simulink model "GSM_TX"  (R2022b)
settings: Solver=ode45  StartTime=0.0  StopTime=inf  RelTol=1e-3  EnableMultiTasking=on
libraries: dsparch4 x2, commanapbnd3 x2
settings Model: Creator=Kyrillos  LastModifiedBy=anand
settings SolverCC: AlgebraicLoopSolver=TrustRegion
settings DataIOCC: LimitDataPoints=on  SaveFormat=Array  InspectSignalLogs=on  ReturnWorkspaceOutputs=off
settings OptimizationCC: LifeSpan=inf
settings DebuggingCC: SolverPrmCheckMsg=warning  UnconnectedInputMsg=warning  UnconnectedOutputMsg=warning  UnconnectedLineMsg=warning  SFUnexpectedBacktrackingDiag=warning  SFNoUnconditionalDefaultTransitionDiag=warning  SFExecutionAtInitializationDiag=none  SFMachineParentedDataDiag=warning  ArithmeticOperatorsInVariantConditions=warning
settings HardwareCC: ProdBitPerPointer=32  ProdBitPerSizeT=32  ProdBitPerPtrDiffT=32  ProdLargestAtomicFloat=None  ProdIntDivRoundTo=Undefined  ProdEndianess=Unspecified  ProdWordSize=32  ProdHWDeviceType=32-bit Generic
settings ModelReferenceCC: PropagateSignalLabelsOutOfModel=off
settings SFSimCC: SimUseLocalCustomCode=off  CustomCodeUndefinedFunction=UseInterfaceOnly
settings RTWCC: RTWUseLocalCustomCode=off
settings CodeAppCC: StateflowObjectComments=on
settings GRTTargetCC: TargetLangStandard=C89/C90 (ANSI)
settings ConfigComp: CovMetricSettings=dw  CovSaveCumulativeToWorkspaceVar=on  CovSaveSingleToWorkspaceVar=on  CovExternalEMLEnable=off  CovSFcnEnable=off
settings ConfigurationSet: Description=SimMechanics 2G

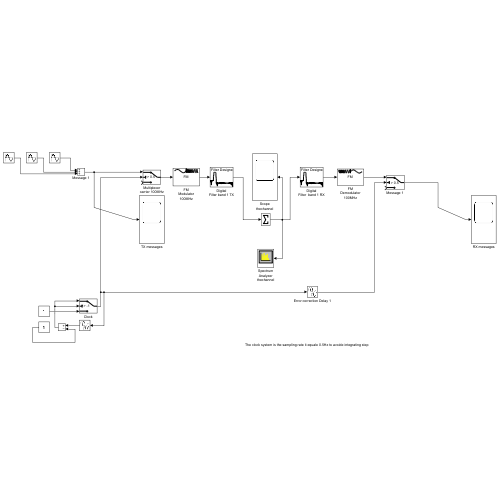
[thumbnail: Simulink's stored preview of the top-level diagram]
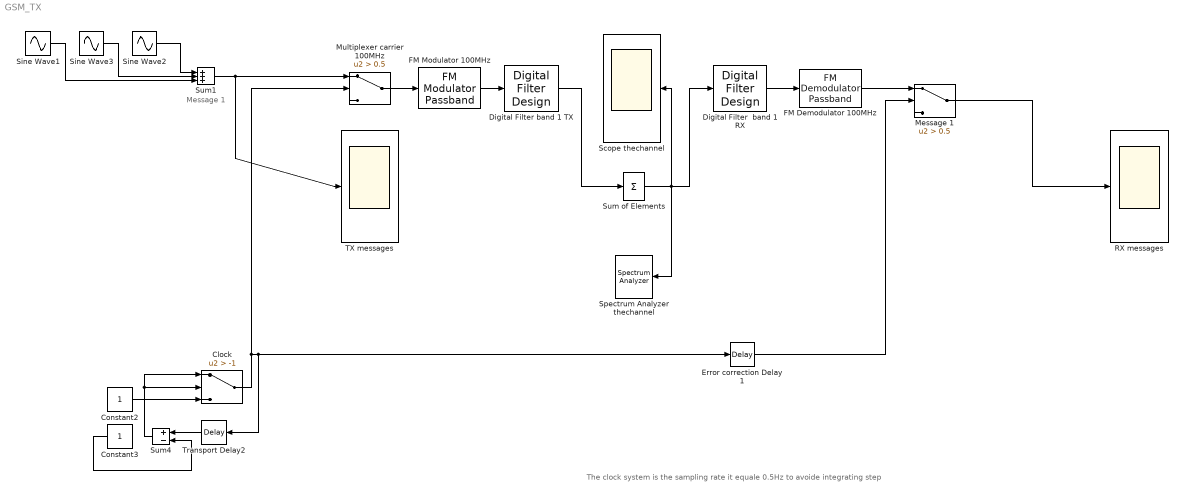
== system GSM_TX ==
  note: The clock system is the sampling rate it equale 0.5Hz to avoide integrating step
  note: Message 1
  Clock : Switch  Criteria=u2 > Threshold  Threshold=-1  SampleTime=0.001  SaturateOnIntegerOverflow=off  InputSameDT=off
  Constant2 : Constant
  Constant3 : Constant
  Digital Filter  band 1 RX : dsparch4/Digital Filter Design  mwdsp_browser_bugfix_var=off
  Digital Filter band 1 TX : dsparch4/Digital Filter Design  mwdsp_browser_bugfix_var=off
  Error correction Delay 1 : TransportDelay  DelayTime=0.3
  FM Demodulator 100MHz : commanapbnd3/FM Demodulator Passband  Fc=100  Ph=0  Kc=0.2  Ho=100
  FM Modulator 100MHz : commanapbnd3/FM Modulator Passband  Fc=100  Ph=0  Kc=0.2
  "Message 1 " : Switch  Criteria=u2 > Threshold  Threshold=0.5  SampleTime=0.001  SaturateOnIntegerOverflow=off  InputSameDT=off
  Multiplexer carrier 100MHz : Switch  Criteria=u2 > Threshold  Threshold=0.5  SampleTime=0.001  SaturateOnIntegerOverflow=off  InputSameDT=off
  RX messages : Scope
      settings: Priority=3
  Scope thechannel : Scope
      settings: Priority=3
  Sine Wave1 : Sin  Amplitude=10/5  Frequency=10*pi  SampleTime=0.001
  Sine Wave2 : Sin  Amplitude=10  Frequency=2*pi  SampleTime=0.001
  Sine Wave3 : Sin  Amplitude=10/3  Frequency=6*pi  SampleTime=0.001
  Spectrum Analyzer thechannel : SpectrumAnalyzer
  Sum of Elements : Sum  Inputs=+  SampleTime=0.001
  Sum1 : Sum  Inputs=+++
  Sum4 : Sum  Inputs=+-
  TX messages : Scope
      settings: Priority=3
  Transport Delay2 : TransportDelay
  wires:
  Sum1/1 -> Multiplexer carrier 100MHz/1, TX messages/1
  Multiplexer carrier 100MHz/1 -> FM Modulator 100MHz/1
  Digital Filter  band 1 RX/1 -> FM Demodulator 100MHz/1
  Sum of Elements/1 -> Spectrum Analyzer thechannel/1, Digital Filter  band 1 RX/1, Scope thechannel/1
  Sine Wave2/1 -> Sum1/1
  Sine Wave3/1 -> Sum1/2
  Sine Wave1/1 -> Sum1/3
  Digital Filter band 1 TX/1 -> Sum of Elements/1
  FM Modulator 100MHz/1 -> Digital Filter band 1 TX/1
  FM Demodulator 100MHz/1 -> "Message 1 "/1
  Sum4/1 -> Clock/1, Clock/2
  Constant3/1 -> Sum4/2
  Transport Delay2/1 -> Sum4/1
  Constant2/1 -> Clock/3
  Clock/1 -> Error correction Delay 1/1, Transport Delay2/1, Multiplexer carrier 100MHz/2
  Error correction Delay 1/1 -> "Message 1 "/2
  "Message 1 "/1 -> RX messages/1
